simulink subsystem "Subsystem_last"  (R2025b)
settings: Solver=VariableStepAuto  StartTime=0.0  StopTime=10.0  RelTol=1e-3
model mask{Waterlevel_1=275, proces=0, Diameter=24.5, Max_cap_1=300, Duration=60*1, Flowrate=1, BurstStart=60, BurstFlow=20, BurstDur=60, rain_start=0, station_order=0, flip_order=off, RainSwitch_S1=on, EnableBurst=on}
  mask prompts: Waterlevel_1 "Initial water level:"; proces "Processing rate (liters/minute):"; Max_cap_1 "Max capacity:"; Duration "Duration (sec):"; Flowrate "Flowrate (liters/min)"; BurstStart "Burst start:"; BurstFlow "Burst flow:"; BurstDur "Burst duration:"; rain_start "Rain start (sec):"; station_order "Station order:"; flip_order "Flip order"; RainSwitch_S1 "Set rain On/Off"; EnableBurst "Enable cloud burst"
settings Model: Creator=klump  LastModifiedBy=klump

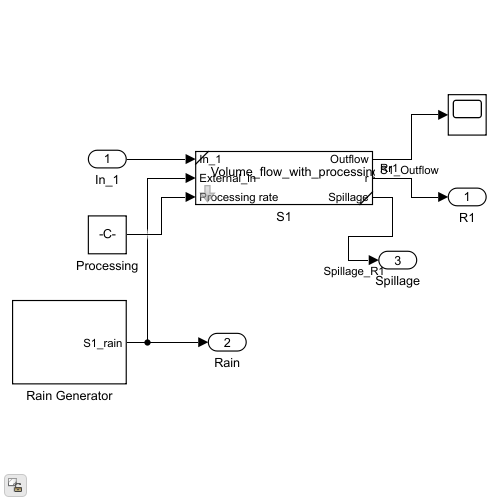
[thumbnail: Simulink's stored preview of the top-level diagram]
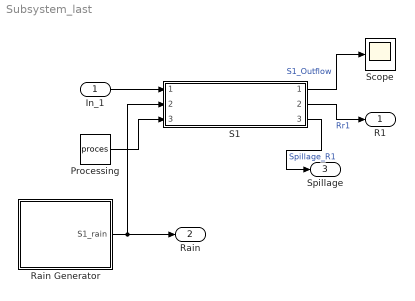
== system Subsystem_last ==
  In_1 : Inport
  Processing : Constant  Value=proces
  Rain Generator : Subsystem
  S1 : Subsystem  ReferencedSubsystem=Volume_flow_with_processing  InitialCondition=Waterlevel_1  Max_cap=Max_cap_1  Diameter=Diameter
  Scope : Scope
      settings: ActiveDisplayYMinimum=0.073333333333333334  ActiveDisplayYMaximum=0.093333333333333324  DataLoggingVariableName=ScopeData25
  R1 : Outport
  Rain : Outport  Port=2
  Spillage : Outport  Port=3
  wires:
  In_1/1 -> S1/1
  Processing/1 -> S1/3
  S1/2 -> R1/1  "Rr1"
  S1/1 -> Scope/1  "S1_Outflow"
  Rain Generator/1(S1_rain) -> S1/2, Rain/1
  S1/3 -> Spillage/1  "Spillage_R1"

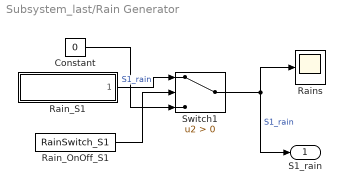
== system Subsystem_last/Rain Generator ==
  Constant : Constant  Value=0
  Rain_OnOff_S1 : Constant  Value=RainSwitch_S1
  Rain_S1 : Subsystem  ReferencedSubsystem=Rain  Duration=Duration  Flowrate=Flowrate  BurstStart=BurstStart  BurstFlow=BurstFlow  BurstDur=BurstDur  flip_order=off  rain_start=rain_start  station_order=station_order  EnableBurst=on
  Rains : Scope
      settings: ActiveDisplayYMinimum=-1  ActiveDisplayYMaximum=1  DataLoggingVariableName=ScopeData2
  Switch1 : Switch  Criteria=u2 > Threshold  SaturateOnIntegerOverflow=off  InputSameDT=off
  S1_rain : Outport
  wires:
  Rain_OnOff_S1/1 -> Switch1/2
  Constant/1 -> Switch1/3
  Switch1/1 -> S1_rain/1, Rains/1  "S1_rain"
  Rain_S1/1 -> Switch1/1  "S1_rain"
